simulink model "Embedded_control_motor_Full"  (R2020b)
settings: Solver=FixedStepAuto  StartTime=0.0  StopTime=10  FixedStep=0.02  RelTol=1e-3  EnableMultiTasking=on
undefined symbols (not defined in the file): DiscIntNeverNeededParam
libraries: arduinolib x4, simulink x1
settings Model: SILPILModeSetting=veronly  EnablePacing=on  ExtModeTrigDuration=2  Creator=Jezz  LastModifiedBy=helve
settings OptimizationCC: EnhancedBackFolding=on  PassReuseOutputArgsAs=Individual arguments  ZeroExternalMemoryAtStartup=off  ZeroInternalMemoryAtStartup=off  MaxStackSize=64  OptimizeBlockOrder=speed  DifferentSizesBufferReuse=on  OptimizationCustomize=off  EfficientTunableParamExpr=on
settings DebuggingCC: ParameterTunabilityLossMsg=error
settings HardwareCC: ProdBitPerPointer=32  ProdBitPerSizeT=32  ProdBitPerPtrDiffT=32  ProdLargestAtomicInteger=Long  ProdLargestAtomicFloat=Double  ProdWordSize=32  ProdHWDeviceType=ARM Compatible->ARM Cortex
settings SFSimCC: MATLABDynamicMemAlloc=off
settings RTWCC: Description=Embedded Coder  SystemTargetFile=ert.tlc  HardwareBoard=Arduino Nano 33 IoT  TemplateMakefile=ert_default_tmf  Toolchain=Arduino ARM  BuildConfiguration=Faster Runs
settings CodeAppCC: ForceParamTrailComments=on  IgnoreCustomStorageClasses=off  OperatorAnnotations=on  SimulinkDataObjDesc=on  SFDataObjDesc=on  InsertBlockDesc=on
settings ERTTargetCC: SupportContinuousTime=on  SupportVariableSizeSignals=on  ExtModeTransport=3  ExtModeStaticAllocSize=8192  ExtModeMexFile=ext_xcp  ExtModeIntrfLevel=Level2 - Open

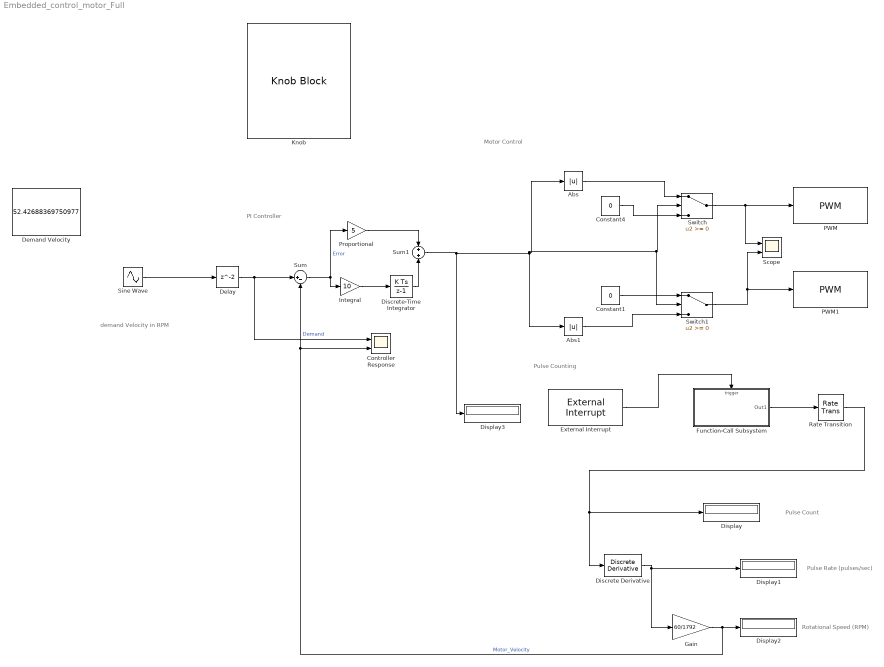
== system Embedded_control_motor_Full ==
  note: demand Velocity in RPM
  note: Pulse Counting
  note: Motor Control
  note: Pulse Rate (pulses/sec)
  note: Pulse Count
  note: Rotational Speed (RPM)
  note: PI Controller
  Abs : Abs
  Abs1 : Abs
  Constant1 : Constant  Value=0  OutDataTypeStr=uint8  SampleTime=-1
  Constant4 : Constant  Value=0  OutDataTypeStr=uint8  SampleTime=-1
  Controller Response : Scope  NumInputPorts=2
  Delay : Delay
  Demand Velocity : Constant  Value=52.42688369750977
  Discrete Derivative : simulink/Discrete/Discrete Derivative  gainval=1.0  ICPrevScaledInput=0.0  OutMin=[]  OutMax=[]  OutDataType=fixdt(1, 16)  OutScaling=2^-10  DoSatur=off
  Discrete-Time Integrator : DiscreteIntegrator  SampleTime=-1  ICPrevOutput=DiscIntNeverNeededParam  ICPrevScaledInput=DiscIntNeverNeededParam
  Display{,1..3} (4 alike) : Display
  External Interrupt : arduinolib/External Interrupt  Pin=2  PullUp=off  Mode=RISING  InterruptSimulationInput=off
      settings: SourceProductBaseCode=ARDUINO
  Function-Call Subsystem : Subsystem  TreatAsAtomicUnit=on
  Gain : Gain  Gain=60/1792
  Integral : Gain  Gain=10
  Knob : KnobBlock  ScaleMax=75
  PWM : arduinolib/PWM  pinNumber=10  frequencyType=Default  desiredFrequency=500  achievableFrequency=500
  PWM1 : arduinolib/PWM  pinNumber=11  frequencyType=Default  desiredFrequency=500  achievableFrequency=500
  Proportional : Gain  Gain=5
  Rate Transition : RateTransition  Deterministic=off
  Scope : Scope  NumInputPorts=2
  Sine Wave : Sin  Amplitude=52  SampleTime=0
  Sum : Sum  Inputs=|+-
  Sum1 : Sum  Inputs=+|+
  Switch : Switch
  Switch1 : Switch
  wires:
  Abs/1 -> Switch/1
  Constant4/1 -> Switch/3
  Switch/1 -> Scope/1, PWM/1
  Abs1/1 -> Switch1/3
  Constant1/1 -> Switch1/1
  Switch1/1 -> PWM1/1, Scope/2
  Rate Transition/1 -> Discrete Derivative/1, Display/1
  External Interrupt/1 -> Function-Call Subsystem/Trigger
  Discrete Derivative/1 -> Gain/1, Display1/1
  Function-Call Subsystem/1(Out1) -> Rate Transition/1
  Discrete-Time Integrator/1 -> Sum1/2
  Integral/1 -> Discrete-Time Integrator/1
  Sum/1 -> Proportional/1, Integral/1  "Error"
  Delay/1 -> Controller Response/1, Sum/1  "Demand"
  Gain/1 -> Controller Response/2, Sum/2, Display2/1  "Motor_Velocity"
  Proportional/1 -> Sum1/1
  Sum1/1 -> Switch1/2, Switch/2, Abs/1, Abs1/1, Display3/1
  Sine Wave/1 -> Delay/1

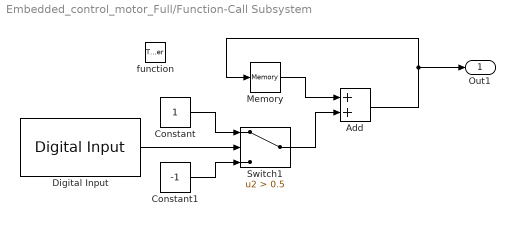
== system Embedded_control_motor_Full/Function-Call Subsystem ==
  function : TriggerPort  TriggerType=function-call  VariantControl=Variant
  Add : Sum
  Constant : Constant  SampleTime=-1
  Constant1 : Constant  Value=-1  SampleTime=-1
  Digital Input : arduinolib/Digital Input  pinNumber=3  mode=Default  Direction=input  SampleTime=-1  blockPlatform=arduino
  Memory : Memory  InheritSampleTime=on
  Switch1 : Switch  Criteria=u2 > Threshold  Threshold=0.5
  Out1 : Outport
  wires:
  Constant/1 -> Switch1/1
  Memory/1 -> Add/1
  Add/1 -> Memory/1, Out1/1
  Digital Input/1 -> Switch1/2
  Constant1/1 -> Switch1/3
  Switch1/1 -> Add/2
